simulink model "Lung Model"  (R2024b)
settings: Solver=VariableStepAuto  StartTime=0.0  StopTime=60  RelTol=1e-3  AbsTol=1e-3
values from neighbouring files (symbols this model uses):
  RbA = 0.082    [Lung Model.m]
  Rtb = 0.212    [Lung Model.m]
  Rtube = 4.0    (= 4)    [Lung Model.m]
libraries: fl_lib x11, nesl_utility x3, cstblocks x2
settings Model: Creator=Deniz  LastModifiedBy=Deniz
settings SolverCC: AutoScaleAbsTol=off  AlgebraicLoopSolver=TrustRegion  MaxZcPerStep=1
settings DebuggingCC: UnconnectedInputMsg=warning  UnconnectedOutputMsg=warning  UnconnectedLineMsg=warning  SymbolicDimsDataTypeCodeGenerationDiagnostic=none
settings ModelReferenceCC: EnableRefExpFcnMdlSchedulingChecks=on
settings SFSimCC: CustomCodeUndefinedFunction=UseInterfaceOnly
settings RTWCC: GPUComputeCapability=3.5  DLArmComputeVersion=19.05
settings SimscapeCC: SimscapeLogType=all  SimscapeLogSimulationStatistics=on  SimscapeLogDataHistory=10000

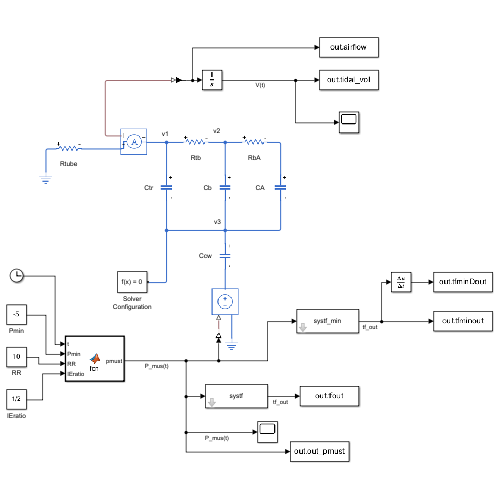
[thumbnail: Simulink's stored preview of the top-level diagram]
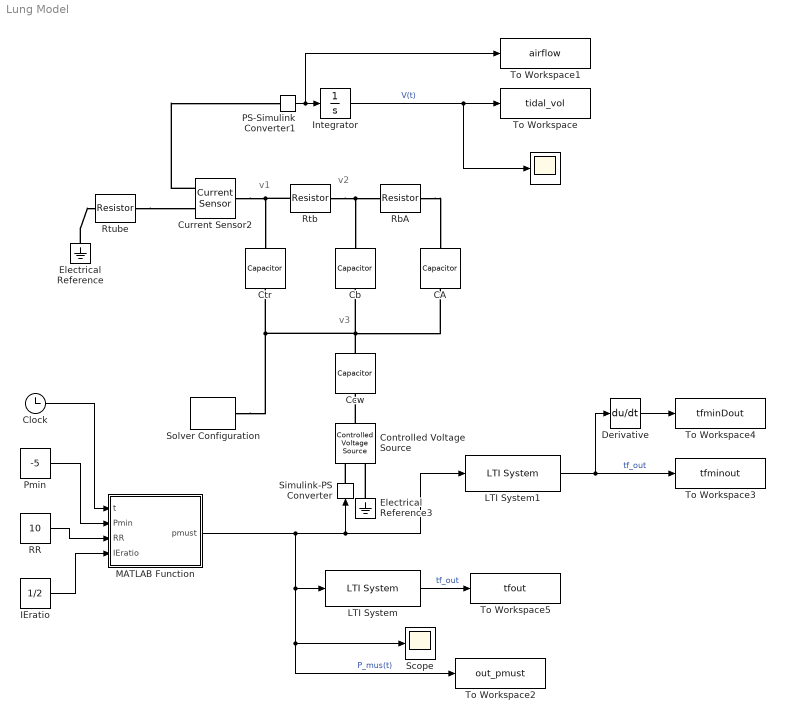
== system Lung Model ==
  note: v1
  note: v2
  note: v3
  "  " : Scope
  CA : fl_lib/Electrical/Electrical Elements/Capacitor  c=CA F  r=0 Ohm  g=0 1/Ohm  i_specify=off  i_priority=None  i=0 A  i_nominal_specify=off  i_nominal_value=1  i_nominal_unit=A  v_specify=off  v_priority=None  v=0 V  v_nominal_specify=off  v_nominal_value=1  v_nominal_unit=V  vc_specify=off  vc_priority=High  vc=0 V  vc_nominal_specify=off  vc_nominal_value=1  vc_nominal_unit=V
  Cb : fl_lib/Electrical/Electrical Elements/Capacitor  c=Cb F  r=0 Ohm  g=0 1/Ohm  i_specify=off  i_priority=None  i=0 A  i_nominal_specify=off  i_nominal_value=1  i_nominal_unit=A  v_specify=off  v_priority=None  v=0 V  v_nominal_specify=off  v_nominal_value=1  v_nominal_unit=V  vc_specify=off  vc_priority=High  vc=0 V  vc_nominal_specify=off  vc_nominal_value=1  vc_nominal_unit=V
  Ccw : fl_lib/Electrical/Electrical Elements/Capacitor  c=Ccw F  r=0 Ohm  g=0 1/Ohm  i_specify=off  i_priority=None  i=0 A  i_nominal_specify=off  i_nominal_value=1  i_nominal_unit=A  v_specify=off  v_priority=None  v=0 V  v_nominal_specify=off  v_nominal_value=1  v_nominal_unit=V  vc_specify=off  vc_priority=High  vc=0 V  vc_nominal_specify=off  vc_nominal_value=1  vc_nominal_unit=V
  Clock : Clock
  Controlled Voltage Source : fl_lib/Electrical/Electrical Sources/Controlled Voltage Source
  Ctr : fl_lib/Electrical/Electrical Elements/Capacitor  c=Ctr F  r=0 Ohm  g=0 1/Ohm  i_specify=off  i_priority=None  i=0 A  i_nominal_specify=off  i_nominal_value=1  i_nominal_unit=A  v_specify=off  v_priority=None  v=0 V  v_nominal_specify=off  v_nominal_value=1  v_nominal_unit=V  vc_specify=off  vc_priority=High  vc=0 V  vc_nominal_specify=off  vc_nominal_value=1  vc_nominal_unit=V
  Current Sensor2 : fl_lib/Electrical/Electrical Sensors/Current Sensor
  Derivative : Derivative
  Electrical Reference : fl_lib/Electrical/Electrical Elements/Electrical Reference
  Electrical Reference3 : fl_lib/Electrical/Electrical Elements/Electrical Reference
  IEratio : Constant  Value=1/2
  Integrator : Integrator
  LTI System : cstblocks/LTI System  sys=systf  IC=[]  PadeOrder=0
  LTI System1 : cstblocks/LTI System  sys=systf_min  IC=[]  PadeOrder=0
  MATLAB Function : MATLAB Function  TreatAsAtomicUnit=on
  PS-Simulink Converter1 : nesl_utility/PS-Simulink Converter  PhysicalDomain=network_engine_domain  SubClassName=ps_output  LeftPortType=input  RightPortType=output  PseudoPeriodic=off  Frequencies=[]  VectorFormat=inherit  Unit=inherit  AffineConversion=off
  Pmin : Constant  Value=-5
  RR : Constant  Value=10
  RbA : fl_lib/Electrical/Electrical Elements/Resistor  R=RbA Ohm  i_specify=off  i_priority=None  i=0 A  i_nominal_specify=off  i_nominal_value=1  i_nominal_unit=A  v_specify=off  v_priority=None  v=0 V  v_nominal_specify=off  v_nominal_value=1  v_nominal_unit=V
  Rtb : fl_lib/Electrical/Electrical Elements/Resistor  R=Rtb Ohm  i_specify=off  i_priority=None  i=0 A  i_nominal_specify=off  i_nominal_value=1  i_nominal_unit=A  v_specify=off  v_priority=None  v=0 V  v_nominal_specify=off  v_nominal_value=1  v_nominal_unit=V
  Rtube : fl_lib/Electrical/Electrical Elements/Resistor  R=Rtube Ohm  i_specify=off  i_priority=None  i=0 A  i_nominal_specify=off  i_nominal_value=1  i_nominal_unit=A  v_specify=off  v_priority=None  v=0 V  v_nominal_specify=off  v_nominal_value=1  v_nominal_unit=V
  Scope : Scope
  Simulink-PS Converter : nesl_utility/Simulink-PS Converter  PhysicalDomain=network_engine_domain  SubClassName=ps_input  LeftPortType=input  RightPortType=output  PseudoPeriodic=off  Frequencies=[]  NoiseDistribution=none  NoiseParameters=[]  Unit=1  AffineConversion=off  FilteringAndDerivatives=provide  SimscapeFilterOrder=1  InputFilterTimeConstant=0.001  UdotUserProvided=0
  Solver Configuration : nesl_utility/Solver Configuration  PhysicalDomain=network_engine_domain  SubClassName=solver  LeftPortType=input  RightPortType=generic  Tones=[]  Harmonics=[]  SimulateNoise=off  Profile=off  UseLocalSampling=off  EnableSwitchedLinearOptims=on  FrequencyDomain=off  UseCCode=off  RelTol=0.001  AbsTol=1e-06  MinStep=1e-09  ToWorkspace=off  RevertToSquareIcSolve=off  NumHomotopyIterations=100  PhasorMode=off  PhasorModeNumHarmonics=1  ConsistencySolver=NEWTON_XTOL_AFTER_FTOL  IndexReductionMethod=DerivativeReplacement  DoDC=off  ResidualTolerance=1e-09  ConsistencyTolSource=GLOBAL  ConsistencyAbsTol=0.001  ConsistencyRelTol=0.001  ConsistencyTolFactor=0.001  UseLocalSolver=on  LocalSolverChoice=NE_BACKWARD_EULER_ADVANCER  ResolveIndetEquations=on  FunctionEvalNumThread=1  LocalSolverSampleTime=0.001  DoFixedCost=off  MaxNonlinIter=3  MaxModeIter=2  ComputeImpulses=off  ImpulseIterations=2  LinearAlgebra=auto  LinearAlgebraNumThread=0  EquationFormulation=NE_TIME_EF  DelaysMemoryBudget=1024  AutomaticFiltering=on  FilteringTimeConstant=0.001  PartitionStorageMethod=AS_NEEDED  PartitionMemoryBudget=1024  PartitionMethod=ROBUST  MultibodyUseLocalSolver=off  MultibodyLocalSolverChoice=ODE1  MultibodyLocalSolverSampleTime=0.001
  To Workspace : ToWorkspace  VariableName=tidal_vol  SaveFormat=Timeseries  SampleTime=-1
  To Workspace1 : ToWorkspace  VariableName=airflow  SaveFormat=Timeseries  SampleTime=-1
  To Workspace2 : ToWorkspace  VariableName=out_pmust  SaveFormat=Timeseries  SampleTime=-1
  To Workspace3 : ToWorkspace  VariableName=tfminout  SaveFormat=Timeseries  SampleTime=-1
  To Workspace4 : ToWorkspace  VariableName=tfminDout  SaveFormat=Timeseries  SampleTime=-1
  To Workspace5 : ToWorkspace  VariableName=tfout  SaveFormat=Timeseries  SampleTime=-1
  wires:
  MATLAB Function/1(pmust) -> LTI System/1, To Workspace2/1, Scope/1, Simulink-PS Converter/1, LTI System1/1  "P_mus(t)"
  Integrator/1 -> To Workspace/1, "  "/1  "V(t)"
  PS-Simulink Converter1/1 -> To Workspace1/1, Integrator/1
  Pmin/1 -> MATLAB Function/2(Pmin)
  IEratio/1 -> MATLAB Function/4(IEratio)
  RR/1 -> MATLAB Function/3(RR)
  Clock/1 -> MATLAB Function/1(t)
  LTI System/1 -> To Workspace5/1  "tf_out"
  Derivative/1 -> To Workspace4/1
  LTI System1/1 -> Derivative/1, To Workspace3/1  "tf_out"
  connections:
  Rtb/LConn1 -- Current Sensor2/LConn1 -- Ctr/LConn1
  Rtb/RConn1 -- RbA/LConn1 -- Cb/LConn1
  RbA/RConn1 -- CA/LConn1
  Ccw/LConn1 -- Cb/RConn1 -- Solver Configuration/RConn1 -- Ctr/RConn1 -- CA/RConn1
  Controlled Voltage Source/LConn1 -- Ccw/RConn1
  Simulink-PS Converter/RConn1 -- Controlled Voltage Source/RConn1
  Electrical Reference/LConn1 -- Rtube/LConn1
  Electrical Reference3/LConn1 -- Controlled Voltage Source/RConn2
  Current Sensor2/RConn1 -- PS-Simulink Converter1/LConn1
  Rtube/RConn1 -- Current Sensor2/RConn2

== matlab function Lung Model/MATLAB Function ==
  data: t input; Pmin input; pmust output; RR input; IEratio input
function pmust = fcn(t, Pmin, RR, IEratio)

y = 0;

T = 60/RR;
TI = T*IEratio/(1+IEratio);
TE = T - TI;
tao = TE/10;

tmod = mod(t, T);

if tmod <= TI
    y = (Pmin)*(T*tmod - tmod^2)/(TI*TE);
elseif tmod > TI
    y = (Pmin)*(exp( -(tmod-TI)/tao ) - exp(-TE/tao) )/(1 - exp(-TE/tao));
end

pmust = y;
